simulink model "reduced_pp"  (R2018a)
settings: Solver=VariableStepAuto  StartTime=0.0  StopTime=10.0  RelTol=1e-3
undefined symbols (not defined in the file or in its folder): DiscIntNeverNeededParam
libraries: simulink x24
settings Model: Creator=ishaf  LastModifiedBy=ishaf

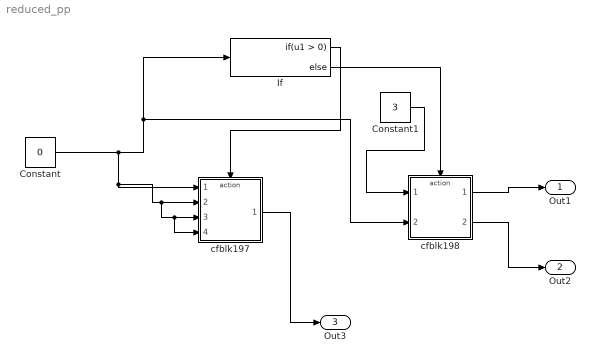
== system reduced_pp ==
  Constant : Constant  Value=0
  Constant1 : Constant  Value=3
  If : If
  cfblk197 : Subsystem  TreatAsAtomicUnit=on
  cfblk198 : Subsystem  TreatAsAtomicUnit=on
  Out1 : Outport
  Out2 : Outport  Port=2
  Out3 : Outport  Port=3
  wires:
  cfblk197/1(cfblk2) -> Out3/1
  Constant/1 -> cfblk197/4(cfblk16), cfblk197/3(cfblk15), cfblk197/2(cfblk14), cfblk197/1(cfblk1), cfblk198/2(cfblk11), If/1
  Constant1/1 -> cfblk198/1(cfblk1)
  cfblk198/1(cfblk2) -> Out1/1
  cfblk198/2(cfblk12) -> Out2/1
  If/1 -> cfblk197/Action
  If/2 -> cfblk198/Action

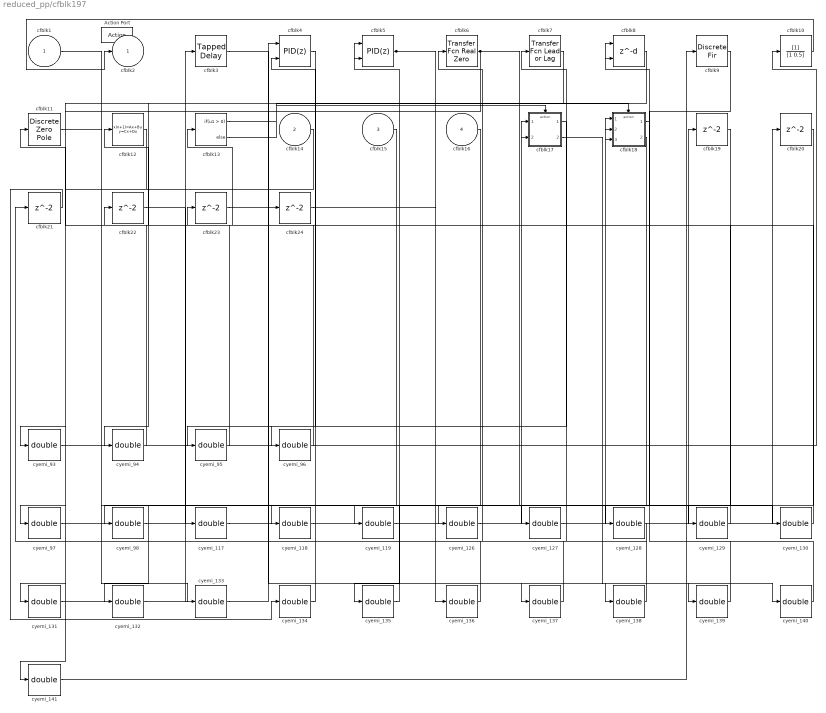
== system reduced_pp/cfblk197 ==
  cfblk1 : Inport
  cfblk14 : Inport  Port=2
  cfblk15 : Inport  Port=3
  cfblk16 : Inport  Port=4
  Action Port : ActionPort  ActionType=then
  cfblk10 : DiscreteFilter
  cfblk11 : DiscreteZeroPole  Poles=[0 0.5]  Gain=1  SampleTime=-1
  cfblk12 : DiscreteStateSpace  SampleTime=-1
  cfblk13 : If  SampleTime=1
  cfblk17 : Subsystem  TreatAsAtomicUnit=on
  cfblk18 : Subsystem  TreatAsAtomicUnit=on
  cfblk{19..24} (6 alike) : Delay
  cfblk3 : simulink/Discrete/Tapped Delay  vinit=0.0  samptime=-1  NumDelays=1  DelayOrder=Oldest  includeCurrent=off
  cfblk4 : simulink/Continuous/PID Controller (2DOF)  Controller=PID  TimeDomain=Discrete-time  SampleTime=-1  IntegratorMethod=Forward Euler  FilterMethod=Forward Euler  Form=Parallel  UseFilter=on  ControllerParametersSource=internal  P=1  I=1  D=0  N=100  b=1  c=1  InitialConditionSource=internal  InitialConditionForIntegrator=0  InitialConditionForFilter=0  ExternalReset=none  LimitOutput=off  UpperSaturationLimit=inf  LowerSaturationLimit=-inf  LinearizeAsGain=off  AntiWindupMode=none  Kb=1  TrackingMode=off  Kt=1  PParamMin=[]  PParamMax=[]  IParamMin=[]  IParamMax=[]  DParamMin=[]  DParamMax=[]  NParamMin=[]  NParamMax=[]  bParamMin=[]  bParamMax=[]  cParamMin=[]  cParamMax=[]  KbParamMin=[]  KbParamMax=[]  KtParamMin=[]  KtParamMax=[]  POutMin=[]  POutMax=[]  IOutMin=[]  IOutMax=[]  DOutMin=[]  DOutMax=[]  NOutMin=[]  NOutMax=[]  bOutMin=[]  bOutMax=[]  cOutMin=[]  cOutMax=[]  KbOutMin=[]  KbOutMax=[]  KtOutMin=[]  KtOutMax=[]  IntegratorOutMin=[]  IntegratorOutMax=[]  FilterOutMin=[]  FilterOutMax=[]  SumOutMin=[]  SumOutMax=[]  Sum1OutMin=[]  Sum1OutMax=[]  Sum2OutMin=[]  Sum2OutMax=[]  Sum3OutMin=[]  Sum3OutMax=[]  SumI1OutMin=[]  SumI1OutMax=[]  SumI2OutMin=[]  SumI2OutMax=[]  SumI3OutMin=[]  SumI3OutMax=[]  SumDOutMin=[]  SumDOutMax=[]  SaturationOutMin=[]  SaturationOutMax=[]  IntegratorContinuousStateAttributes=''  IntegratorStateMustResolveToSignalObject=off  IntegratorRTWStateStorageClass=Auto  FilterContinuousStateAttributes=''  FilterStateMustResolveToSignalObject=off  FilterRTWStateStorageClass=Auto  DifferentiatorICPrevScaledInput=0  DifferentiatorOutMin=[]  DifferentiatorOutMax=[]  FilterDiffOutCoefMin=[]  FilterDiffOutCoefMax=[]  SumDenOutMin=[]  SumDenOutMax=[]  SumNumOutMin=[]  SumNumOutMax=[]  ReciprocalOutMin=[]  ReciprocalOutMax=[]  DivideOutMin=[]  DivideOutMax=[]  TunerSelectOption=Transfer Function Based (PID Tuner App)
  cfblk5 : simulink/Continuous/PID Controller (2DOF)  Controller=PID  TimeDomain=Discrete-time  SampleTime=-1  IntegratorMethod=Forward Euler  FilterMethod=Forward Euler  Form=Parallel  UseFilter=on  ControllerParametersSource=internal  P=1  I=1  D=0  N=100  b=1  c=1  InitialConditionSource=internal  InitialConditionForIntegrator=0  InitialConditionForFilter=0  ExternalReset=none  LimitOutput=off  UpperSaturationLimit=inf  LowerSaturationLimit=-inf  LinearizeAsGain=off  AntiWindupMode=none  Kb=1  TrackingMode=off  Kt=1  PParamMin=[]  PParamMax=[]  IParamMin=[]  IParamMax=[]  DParamMin=[]  DParamMax=[]  NParamMin=[]  NParamMax=[]  bParamMin=[]  bParamMax=[]  cParamMin=[]  cParamMax=[]  KbParamMin=[]  KbParamMax=[]  KtParamMin=[]  KtParamMax=[]  POutMin=[]  POutMax=[]  IOutMin=[]  IOutMax=[]  DOutMin=[]  DOutMax=[]  NOutMin=[]  NOutMax=[]  bOutMin=[]  bOutMax=[]  cOutMin=[]  cOutMax=[]  KbOutMin=[]  KbOutMax=[]  KtOutMin=[]  KtOutMax=[]  IntegratorOutMin=[]  IntegratorOutMax=[]  FilterOutMin=[]  FilterOutMax=[]  SumOutMin=[]  SumOutMax=[]  Sum1OutMin=[]  Sum1OutMax=[]  Sum2OutMin=[]  Sum2OutMax=[]  Sum3OutMin=[]  Sum3OutMax=[]  SumI1OutMin=[]  SumI1OutMax=[]  SumI2OutMin=[]  SumI2OutMax=[]  SumI3OutMin=[]  SumI3OutMax=[]  SumDOutMin=[]  SumDOutMax=[]  SaturationOutMin=[]  SaturationOutMax=[]  IntegratorContinuousStateAttributes=''  IntegratorStateMustResolveToSignalObject=off  IntegratorRTWStateStorageClass=Auto  FilterContinuousStateAttributes=''  FilterStateMustResolveToSignalObject=off  FilterRTWStateStorageClass=Auto  DifferentiatorICPrevScaledInput=0  DifferentiatorOutMin=[]  DifferentiatorOutMax=[]  FilterDiffOutCoefMin=[]  FilterDiffOutCoefMax=[]  SumDenOutMin=[]  SumDenOutMax=[]  SumNumOutMin=[]  SumNumOutMax=[]  ReciprocalOutMin=[]  ReciprocalOutMax=[]  DivideOutMin=[]  DivideOutMax=[]  TunerSelectOption=Transfer Function Based (PID Tuner App)
  cfblk6 : simulink/Discrete/Transfer Fcn Real Zero  ZeroZ=0.75  ICPrevInput=0.0  DoSatur=off
      settings: SourceProductName=Simulink  SourceProductBaseCode=SL
  cfblk7 : simulink/Discrete/Transfer Fcn Lead or Lag  PoleZ=0.95  ZeroZ=0.75  ICPrevOutput=0.0  ICPrevInput=0.0  DoSatur=off
      settings: SourceProductName=Simulink  SourceProductBaseCode=SL
  cfblk8 : Delay  DelayLengthSource=Input port
      settings: InputPortMap=u0,p1
  cfblk9 : DiscreteFir
  cyemi_{93..98,117..119,126..141} (25 alike) : DataTypeConversion  OutDataTypeStr=double
  cfblk2 : Outport
  wires:
  cfblk5/1 -> cyemi_129/1, cyemi_137/1
  cfblk6/1 -> cyemi_130/1, cyemi_131/1
  cfblk10/1 -> cfblk2/1
  cfblk13/1 -> cfblk17/Action
  cfblk13/2 -> cfblk18/Action
  cyemi_93/1 -> cfblk10/1
  cfblk14/1 -> cyemi_93/1
  cyemi_94/1 -> cfblk11/1
  cfblk8/1 -> cyemi_94/1
  cyemi_95/1 -> cfblk12/1
  cfblk17/1(cfblk2) -> cyemi_95/1
  cyemi_96/1 -> cfblk13/1
  cfblk4/1 -> cyemi_96/1
  cyemi_97/1 -> cfblk17/1(cfblk1)
  cfblk7/1 -> cyemi_97/1
  cyemi_98/1 -> cfblk17/2(cfblk16)
  cfblk19/1 -> cyemi_98/1
  cyemi_117/1 -> cfblk18/1(cfblk1)
  cfblk22/1 -> cyemi_117/1
  cyemi_118/1 -> cfblk18/2(cfblk9)
  cfblk20/1 -> cyemi_118/1
  cyemi_119/1 -> cfblk18/3(cfblk10)
  cfblk15/1 -> cyemi_119/1
  cyemi_126/1 -> cfblk19/1
  cfblk9/1 -> cyemi_126/1
  cyemi_127/1 -> cfblk20/1
  cfblk11/1 -> cyemi_127/1
  cyemi_128/1 -> cfblk21/1
  cfblk18/1(cfblk2) -> cyemi_128/1
  cyemi_129/1 -> cfblk22/1
  cyemi_130/1 -> cfblk23/1
  cyemi_131/1 -> cfblk24/1
  cyemi_132/1 -> cfblk3/1
  cfblk16/1 -> cyemi_132/1
  cyemi_133/1 -> cfblk4/1
  cfblk1/1 -> cyemi_133/1
  cyemi_134/1 -> cfblk4/2
  cfblk21/1 -> cyemi_134/1
  cyemi_135/1 -> cfblk5/1
  cfblk18/2(cfblk11) -> cyemi_135/1
  cyemi_136/1 -> cfblk5/2
  cfblk24/1 -> cyemi_136/1
  cyemi_137/1 -> cfblk6/1
  cyemi_138/1 -> cfblk7/1
  cfblk3/1 -> cyemi_138/1
  cyemi_139/1 -> cfblk8/1
  cfblk23/1 -> cyemi_139/1
  cyemi_140/1 -> cfblk8/2
  cfblk17/2(cfblk17) -> cyemi_140/1
  cyemi_141/1 -> cfblk9/1
  cfblk12/1 -> cyemi_141/1

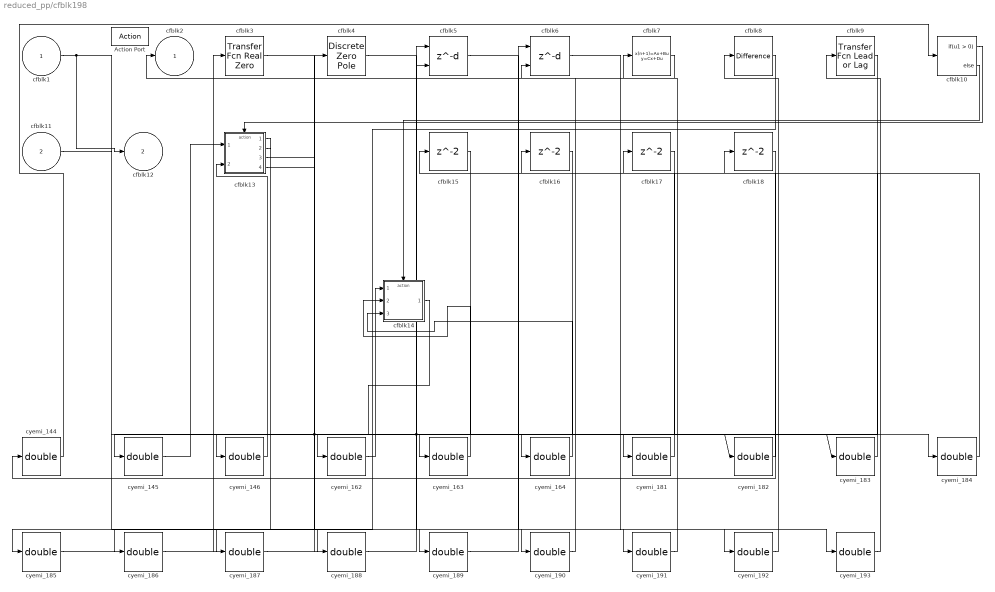
== system reduced_pp/cfblk198 ==
  cfblk1 : Inport
  cfblk11 : Inport  Port=2
  Action Port : ActionPort  ActionType=else
  cfblk10 : If  SampleTime=1
  cfblk13 : Subsystem  TreatAsAtomicUnit=on
  cfblk14 : Subsystem  TreatAsAtomicUnit=on
  cfblk{15..18} (4 alike) : Delay
  cfblk3 : simulink/Discrete/Transfer Fcn Real Zero  ZeroZ=0.75  ICPrevInput=0.0  DoSatur=off
      settings: SourceProductName=Simulink  SourceProductBaseCode=SL
  cfblk4 : DiscreteZeroPole  Poles=[0 0.5]  Gain=1  SampleTime=-1
  cfblk5 : Delay  DelayLengthSource=Input port
      settings: InputPortMap=u0,p1
  cfblk6 : Delay  DelayLengthSource=Input port
      settings: InputPortMap=u0,p1
  cfblk7 : DiscreteStateSpace  SampleTime=-1
  cfblk8 : simulink/Discrete/Difference  ICPrevInput=0.0  OutMin=[]  OutMax=[]  OutDataTypeStr=Inherit: Inherit via back propagation  OutDataType=fixdt(1, 16)  OutScaling=2^-10  DoSatur=off
  cfblk9 : simulink/Discrete/Transfer Fcn Lead or Lag  PoleZ=0.95  ZeroZ=0.75  ICPrevOutput=0.0  ICPrevInput=0.0  DoSatur=off
      settings: SourceProductName=Simulink  SourceProductBaseCode=SL
  cyemi_{144..146,162..164,181..193} (19 alike) : DataTypeConversion  OutDataTypeStr=double
  cfblk2 : Outport
  cfblk12 : Outport  Port=2
  wires:
  cfblk3/1 -> cyemi_182/1, cyemi_189/1
  cfblk7/1 -> cfblk2/1
  cfblk1/1 -> cfblk12/1, cyemi_162/1
  cfblk4/1 -> cyemi_183/1, cyemi_191/1
  cfblk10/1 -> cfblk13/Action
  cfblk10/2 -> cfblk14/Action
  cyemi_144/1 -> cfblk10/1
  cfblk18/1 -> cyemi_144/1
  cyemi_145/1 -> cfblk13/1(cfblk1)
  cfblk14/1(cfblk2) -> cyemi_145/1
  cyemi_146/1 -> cfblk13/2(cfblk13)
  cfblk15/1 -> cyemi_146/1
  cyemi_162/1 -> cfblk14/1(cfblk1)
  cyemi_163/1 -> cfblk14/2(cfblk11)
  cfblk17/1 -> cyemi_163/1
  cyemi_164/1 -> cfblk14/3(cfblk12)
  cfblk16/1 -> cyemi_164/1
  cyemi_181/1 -> cfblk15/1
  cfblk9/1 -> cyemi_181/1
  cyemi_182/1 -> cfblk16/1
  cyemi_183/1 -> cfblk17/1
  cyemi_184/1 -> cfblk18/1
  cfblk13/3(cfblk15) -> cyemi_184/1
  cyemi_185/1 -> cfblk3/1
  cfblk13/1(cfblk2) -> cyemi_185/1
  cyemi_186/1 -> cfblk4/1
  cfblk13/2(cfblk14) -> cyemi_186/1
  cyemi_187/1 -> cfblk5/1
  cfblk8/1 -> cyemi_187/1
  cyemi_188/1 -> cfblk5/2
  cfblk11/1 -> cyemi_188/1
  cyemi_189/1 -> cfblk6/1
  cyemi_190/1 -> cfblk6/2
  cfblk13/4(cfblk16) -> cyemi_190/1
  cyemi_191/1 -> cfblk7/1
  cyemi_192/1 -> cfblk8/1
  cfblk6/1 -> cyemi_192/1
  cyemi_193/1 -> cfblk9/1
  cfblk5/1 -> cyemi_193/1

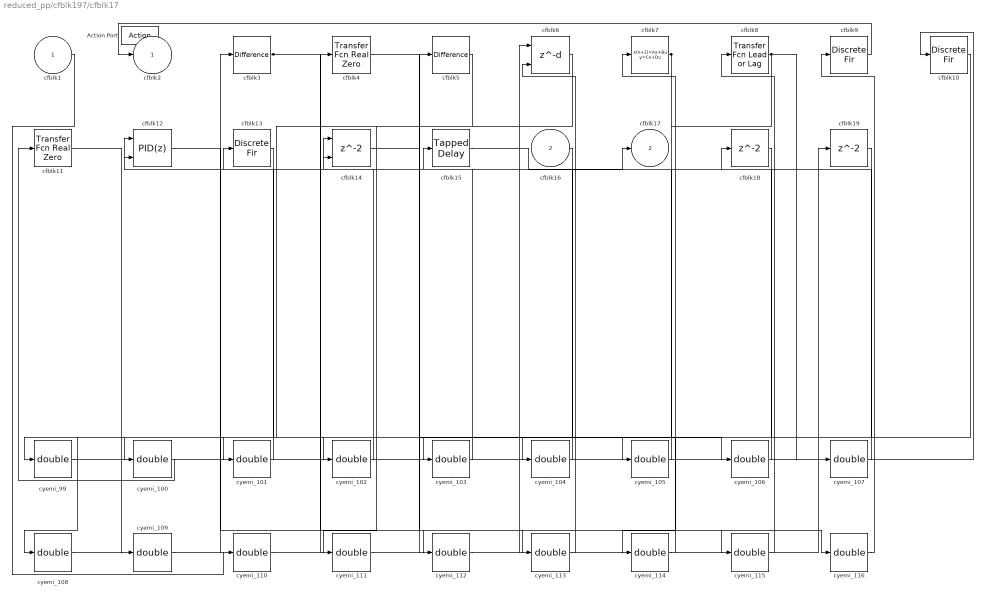
== system reduced_pp/cfblk197/cfblk17 ==
  cfblk1 : Inport
  cfblk16 : Inport  Port=2
  Action Port : ActionPort  ActionType=then
  cfblk10 : DiscreteFir
  cfblk11 : simulink/Discrete/Transfer Fcn Real Zero  ZeroZ=0.75  ICPrevInput=0.0  DoSatur=off
      settings: SourceProductName=Simulink  SourceProductBaseCode=SL
  cfblk12 : simulink/Continuous/PID Controller (2DOF)  Controller=PID  TimeDomain=Discrete-time  SampleTime=-1  IntegratorMethod=Forward Euler  FilterMethod=Forward Euler  Form=Parallel  UseFilter=on  ControllerParametersSource=internal  P=1  I=1  D=0  N=100  b=1  c=1  InitialConditionSource=internal  InitialConditionForIntegrator=0  InitialConditionForFilter=0  ExternalReset=none  LimitOutput=off  UpperSaturationLimit=inf  LowerSaturationLimit=-inf  LinearizeAsGain=off  AntiWindupMode=none  Kb=1  TrackingMode=off  Kt=1  PParamMin=[]  PParamMax=[]  IParamMin=[]  IParamMax=[]  DParamMin=[]  DParamMax=[]  NParamMin=[]  NParamMax=[]  bParamMin=[]  bParamMax=[]  cParamMin=[]  cParamMax=[]  KbParamMin=[]  KbParamMax=[]  KtParamMin=[]  KtParamMax=[]  POutMin=[]  POutMax=[]  IOutMin=[]  IOutMax=[]  DOutMin=[]  DOutMax=[]  NOutMin=[]  NOutMax=[]  bOutMin=[]  bOutMax=[]  cOutMin=[]  cOutMax=[]  KbOutMin=[]  KbOutMax=[]  KtOutMin=[]  KtOutMax=[]  IntegratorOutMin=[]  IntegratorOutMax=[]  FilterOutMin=[]  FilterOutMax=[]  SumOutMin=[]  SumOutMax=[]  Sum1OutMin=[]  Sum1OutMax=[]  Sum2OutMin=[]  Sum2OutMax=[]  Sum3OutMin=[]  Sum3OutMax=[]  SumI1OutMin=[]  SumI1OutMax=[]  SumI2OutMin=[]  SumI2OutMax=[]  SumI3OutMin=[]  SumI3OutMax=[]  SumDOutMin=[]  SumDOutMax=[]  SaturationOutMin=[]  SaturationOutMax=[]  IntegratorContinuousStateAttributes=''  IntegratorStateMustResolveToSignalObject=off  IntegratorRTWStateStorageClass=Auto  FilterContinuousStateAttributes=''  FilterStateMustResolveToSignalObject=off  FilterRTWStateStorageClass=Auto  DifferentiatorICPrevScaledInput=0  DifferentiatorOutMin=[]  DifferentiatorOutMax=[]  FilterDiffOutCoefMin=[]  FilterDiffOutCoefMax=[]  SumDenOutMin=[]  SumDenOutMax=[]  SumNumOutMin=[]  SumNumOutMax=[]  ReciprocalOutMin=[]  ReciprocalOutMax=[]  DivideOutMin=[]  DivideOutMax=[]  TunerSelectOption=Transfer Function Based (PID Tuner App)
  cfblk13 : DiscreteFir
  cfblk14 : Delay  ShowEnablePort=on
      settings: InputPortMap=u0,e6
  cfblk15 : simulink/Discrete/Tapped Delay  vinit=0.0  samptime=-1  NumDelays=1  DelayOrder=Oldest  includeCurrent=off
  cfblk18 : Delay
  cfblk19 : Delay
  cfblk3 : simulink/Discrete/Difference  ICPrevInput=0.0  OutMin=[]  OutMax=[]  OutDataTypeStr=Inherit: Inherit via back propagation  OutDataType=fixdt(1, 16)  OutScaling=2^-10  DoSatur=off
  cfblk4 : simulink/Discrete/Transfer Fcn Real Zero  ZeroZ=0.75  ICPrevInput=0.0  DoSatur=off
      settings: SourceProductName=Simulink  SourceProductBaseCode=SL
  cfblk5 : simulink/Discrete/Difference  ICPrevInput=0.0  OutMin=[]  OutMax=[]  OutDataTypeStr=Inherit: Inherit via back propagation  OutDataType=fixdt(1, 16)  OutScaling=2^-10  DoSatur=off
  cfblk6 : Delay  DelayLengthSource=Input port
      settings: InputPortMap=u0,p1
  cfblk7 : DiscreteStateSpace  SampleTime=-1
  cfblk8 : simulink/Discrete/Transfer Fcn Lead or Lag  PoleZ=0.95  ZeroZ=0.75  ICPrevOutput=0.0  ICPrevInput=0.0  DoSatur=off
      settings: SourceProductName=Simulink  SourceProductBaseCode=SL
  cfblk9 : DiscreteFir
  cyemi_{99..116} (18 alike) : DataTypeConversion  OutDataTypeStr=double
  cfblk2 : Outport
  cfblk17 : Outport  Port=2
  wires:
  cfblk15/1 -> cfblk17/1
  cfblk7/1 -> cyemi_100/1, cyemi_103/1
  cfblk9/1 -> cfblk2/1
  cfblk3/1 -> cyemi_112/1, cyemi_116/1
  cfblk8/1 -> cyemi_105/1, cyemi_107/1
  cyemi_99/1 -> cfblk10/1
  cfblk16/1 -> cyemi_99/1
  cyemi_100/1 -> cfblk11/1
  cyemi_101/1 -> cfblk12/1
  cfblk5/1 -> cyemi_101/1
  cyemi_102/1 -> cfblk12/2
  cfblk18/1 -> cyemi_102/1
  cyemi_103/1 -> cfblk13/1
  cyemi_104/1 -> cfblk14/1
  cfblk10/1 -> cyemi_104/1
  cyemi_105/1 -> cfblk14/2
  cyemi_106/1 -> cfblk15/1
  cfblk14/1 -> cyemi_106/1
  cyemi_107/1 -> cfblk18/1
  cyemi_108/1 -> cfblk19/1
  cfblk13/1 -> cyemi_108/1
  cyemi_109/1 -> cfblk3/1
  cfblk11/1 -> cyemi_109/1
  cyemi_110/1 -> cfblk4/1
  cfblk1/1 -> cyemi_110/1
  cyemi_111/1 -> cfblk5/1
  cfblk6/1 -> cyemi_111/1
  cyemi_112/1 -> cfblk6/1
  cyemi_113/1 -> cfblk6/2
  cfblk4/1 -> cyemi_113/1
  cyemi_114/1 -> cfblk7/1
  cfblk19/1 -> cyemi_114/1
  cyemi_115/1 -> cfblk8/1
  cfblk12/1 -> cyemi_115/1
  cyemi_116/1 -> cfblk9/1

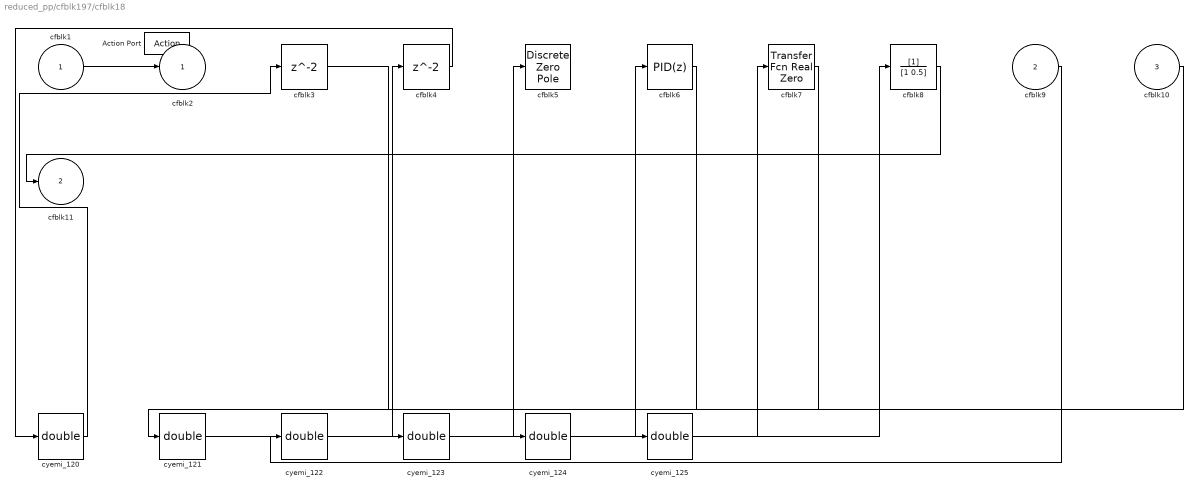
== system reduced_pp/cfblk197/cfblk18 ==
  cfblk1 : Inport
  cfblk9 : Inport  Port=2
  cfblk10 : Inport  Port=3
  Action Port : ActionPort  ActionType=else
  cfblk3 : Delay
  cfblk4 : Delay
  cfblk5 : DiscreteZeroPole  Poles=[0 0.5]  Gain=1  SampleTime=-1
  cfblk6 : simulink/Continuous/PID Controller  Controller=PID  TimeDomain=Discrete-time  SampleTime=-1  IntegratorMethod=Forward Euler  FilterMethod=Forward Euler  Form=Parallel  UseFilter=on  ControllerParametersSource=internal  P=1  I=1  D=0  N=100  InitialConditionSource=internal  InitialConditionForIntegrator=0  InitialConditionForFilter=0  ExternalReset=none  LimitOutput=off  UpperSaturationLimit=inf  LowerSaturationLimit=-inf  LinearizeAsGain=off  AntiWindupMode=none  Kb=1  TrackingMode=off  Kt=1  PParamMin=[]  PParamMax=[]  IParamMin=[]  IParamMax=[]  DParamMin=[]  DParamMax=[]  NParamMin=[]  NParamMax=[]  KbParamMin=[]  KbParamMax=[]  KtParamMin=[]  KtParamMax=[]  POutMin=[]  POutMax=[]  IOutMin=[]  IOutMax=[]  DOutMin=[]  DOutMax=[]  NOutMin=[]  NOutMax=[]  KbOutMin=[]  KbOutMax=[]  KtOutMin=[]  KtOutMax=[]  IntegratorOutMin=[]  IntegratorOutMax=[]  FilterOutMin=[]  FilterOutMax=[]  SumOutMin=[]  SumOutMax=[]  SumI1OutMin=[]  SumI1OutMax=[]  SumI2OutMin=[]  SumI2OutMax=[]  SumI3OutMin=[]  SumI3OutMax=[]  SumDOutMin=[]  SumDOutMax=[]  SaturationOutMin=[]  SaturationOutMax=[]  IntegratorContinuousStateAttributes=''  IntegratorStateMustResolveToSignalObject=off  IntegratorRTWStateStorageClass=Auto  FilterContinuousStateAttributes=''  FilterStateMustResolveToSignalObject=off  FilterRTWStateStorageClass=Auto  DifferentiatorICPrevScaledInput=0  DifferentiatorOutMin=[]  DifferentiatorOutMax=[]  FilterDiffOutCoefMin=[]  FilterDiffOutCoefMax=[]  SumDenOutMin=[]  SumDenOutMax=[]  SumNumOutMin=[]  SumNumOutMax=[]  ReciprocalOutMin=[]  ReciprocalOutMax=[]  DivideOutMin=[]  DivideOutMax=[]  TunerSelectOption=Transfer Function Based (PID Tuner App)
  cfblk7 : simulink/Discrete/Transfer Fcn Real Zero  ZeroZ=0.75  ICPrevInput=0.0  DoSatur=off
      settings: SourceProductName=Simulink  SourceProductBaseCode=SL
  cfblk8 : DiscreteFilter
  cyemi_{120..125} (6 alike) : DataTypeConversion  OutDataTypeStr=double
  cfblk2 : Outport
  cfblk11 : Outport  Port=2
  wires:
  cfblk8/1 -> cfblk11/1
  cfblk1/1 -> cfblk2/1
  cyemi_120/1 -> cfblk3/1
  cfblk4/1 -> cyemi_120/1
  cyemi_121/1 -> cfblk4/1
  cfblk6/1 -> cyemi_121/1
  cyemi_122/1 -> cfblk5/1
  cfblk9/1 -> cyemi_122/1
  cyemi_123/1 -> cfblk6/1
  cfblk10/1 -> cyemi_123/1
  cyemi_124/1 -> cfblk7/1
  cfblk3/1 -> cyemi_124/1
  cyemi_125/1 -> cfblk8/1
  cfblk7/1 -> cyemi_125/1

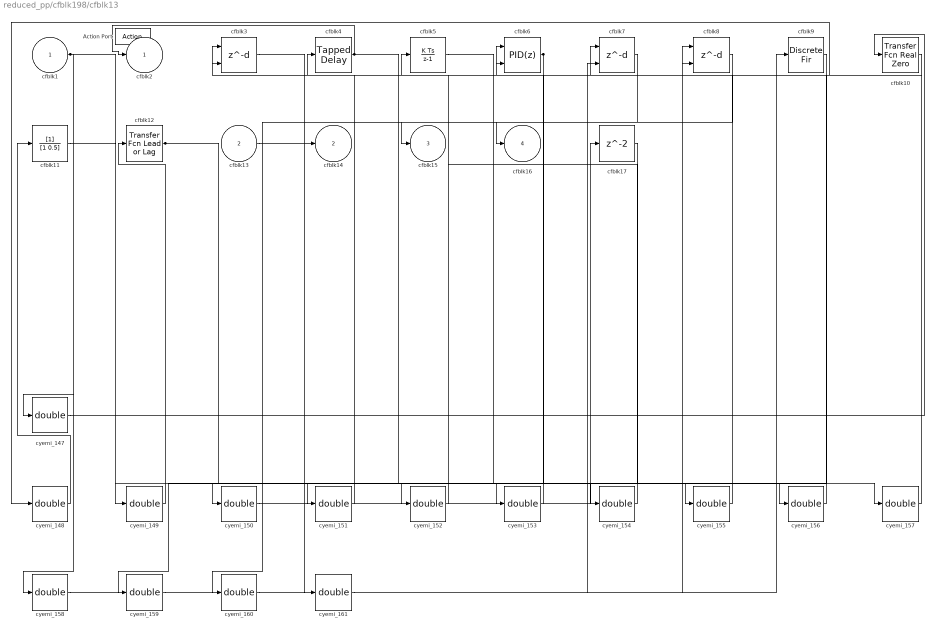
== system reduced_pp/cfblk198/cfblk13 ==
  cfblk1 : Inport
  cfblk13 : Inport  Port=2
  Action Port : ActionPort  ActionType=then
  cfblk10 : simulink/Discrete/Transfer Fcn Real Zero  ZeroZ=0.75  ICPrevInput=0.0  DoSatur=off
      settings: SourceProductName=Simulink  SourceProductBaseCode=SL
  cfblk11 : DiscreteFilter
  cfblk12 : simulink/Discrete/Transfer Fcn Lead or Lag  PoleZ=0.95  ZeroZ=0.75  ICPrevOutput=0.0  ICPrevInput=0.0  DoSatur=off
      settings: SourceProductName=Simulink  SourceProductBaseCode=SL
  cfblk17 : Delay
  cfblk3 : Delay  DelayLengthSource=Input port
      settings: InputPortMap=u0,p1
  cfblk4 : simulink/Discrete/Tapped Delay  vinit=0.0  samptime=-1  NumDelays=1  DelayOrder=Oldest  includeCurrent=off
  cfblk5 : DiscreteIntegrator  SampleTime=-1  ICPrevOutput=DiscIntNeverNeededParam  ICPrevScaledInput=DiscIntNeverNeededParam
  cfblk6 : simulink/Continuous/PID Controller (2DOF)  Controller=PID  TimeDomain=Discrete-time  SampleTime=-1  IntegratorMethod=Forward Euler  FilterMethod=Forward Euler  Form=Parallel  UseFilter=on  ControllerParametersSource=internal  P=1  I=1  D=0  N=100  b=1  c=1  InitialConditionSource=internal  InitialConditionForIntegrator=0  InitialConditionForFilter=0  ExternalReset=none  LimitOutput=off  UpperSaturationLimit=inf  LowerSaturationLimit=-inf  LinearizeAsGain=off  AntiWindupMode=none  Kb=1  TrackingMode=off  Kt=1  PParamMin=[]  PParamMax=[]  IParamMin=[]  IParamMax=[]  DParamMin=[]  DParamMax=[]  NParamMin=[]  NParamMax=[]  bParamMin=[]  bParamMax=[]  cParamMin=[]  cParamMax=[]  KbParamMin=[]  KbParamMax=[]  KtParamMin=[]  KtParamMax=[]  POutMin=[]  POutMax=[]  IOutMin=[]  IOutMax=[]  DOutMin=[]  DOutMax=[]  NOutMin=[]  NOutMax=[]  bOutMin=[]  bOutMax=[]  cOutMin=[]  cOutMax=[]  KbOutMin=[]  KbOutMax=[]  KtOutMin=[]  KtOutMax=[]  IntegratorOutMin=[]  IntegratorOutMax=[]  FilterOutMin=[]  FilterOutMax=[]  SumOutMin=[]  SumOutMax=[]  Sum1OutMin=[]  Sum1OutMax=[]  Sum2OutMin=[]  Sum2OutMax=[]  Sum3OutMin=[]  Sum3OutMax=[]  SumI1OutMin=[]  SumI1OutMax=[]  SumI2OutMin=[]  SumI2OutMax=[]  SumI3OutMin=[]  SumI3OutMax=[]  SumDOutMin=[]  SumDOutMax=[]  SaturationOutMin=[]  SaturationOutMax=[]  IntegratorContinuousStateAttributes=''  IntegratorStateMustResolveToSignalObject=off  IntegratorRTWStateStorageClass=Auto  FilterContinuousStateAttributes=''  FilterStateMustResolveToSignalObject=off  FilterRTWStateStorageClass=Auto  DifferentiatorICPrevScaledInput=0  DifferentiatorOutMin=[]  DifferentiatorOutMax=[]  FilterDiffOutCoefMin=[]  FilterDiffOutCoefMax=[]  SumDenOutMin=[]  SumDenOutMax=[]  SumNumOutMin=[]  SumNumOutMax=[]  ReciprocalOutMin=[]  ReciprocalOutMax=[]  DivideOutMin=[]  DivideOutMax=[]  TunerSelectOption=Transfer Function Based (PID Tuner App)
  cfblk7 : Delay  DelayLengthSource=Input port
      settings: InputPortMap=u0,p1
  cfblk8 : Delay  DelayLengthSource=Input port
      settings: InputPortMap=u0,p1
  cfblk9 : DiscreteFir
  cyemi_{147..161} (15 alike) : DataTypeConversion  OutDataTypeStr=double
  cfblk2 : Outport
  cfblk14 : Outport  Port=2
  cfblk15 : Outport  Port=3
  cfblk16 : Outport  Port=4
  wires:
  cfblk1/1 -> cyemi_147/1, cyemi_155/1, cyemi_158/1
  cfblk4/1 -> cfblk2/1, cyemi_156/1
  cfblk12/1 -> cyemi_154/1, cyemi_161/1
  cfblk13/1 -> cfblk14/1
  cfblk6/1 -> cfblk15/1, cyemi_150/1, cyemi_159/1
  cfblk8/1 -> cfblk16/1
  cyemi_147/1 -> cfblk10/1
  cyemi_148/1 -> cfblk11/1
  cfblk10/1 -> cyemi_148/1
  cyemi_149/1 -> cfblk12/1
  cfblk11/1 -> cyemi_149/1
  cyemi_150/1 -> cfblk17/1
  cyemi_151/1 -> cfblk3/1
  cfblk9/1 -> cyemi_151/1
  cyemi_152/1 -> cfblk3/2
  cfblk17/1 -> cyemi_152/1
  cyemi_153/1 -> cfblk4/1
  cfblk3/1 -> cyemi_153/1
  cyemi_154/1 -> cfblk5/1
  cyemi_155/1 -> cfblk6/1
  cyemi_156/1 -> cfblk6/2
  cyemi_157/1 -> cfblk7/1
  cfblk5/1 -> cyemi_157/1
  cyemi_158/1 -> cfblk7/2
  cyemi_159/1 -> cfblk8/1
  cyemi_160/1 -> cfblk8/2
  cfblk7/1 -> cyemi_160/1
  cyemi_161/1 -> cfblk9/1

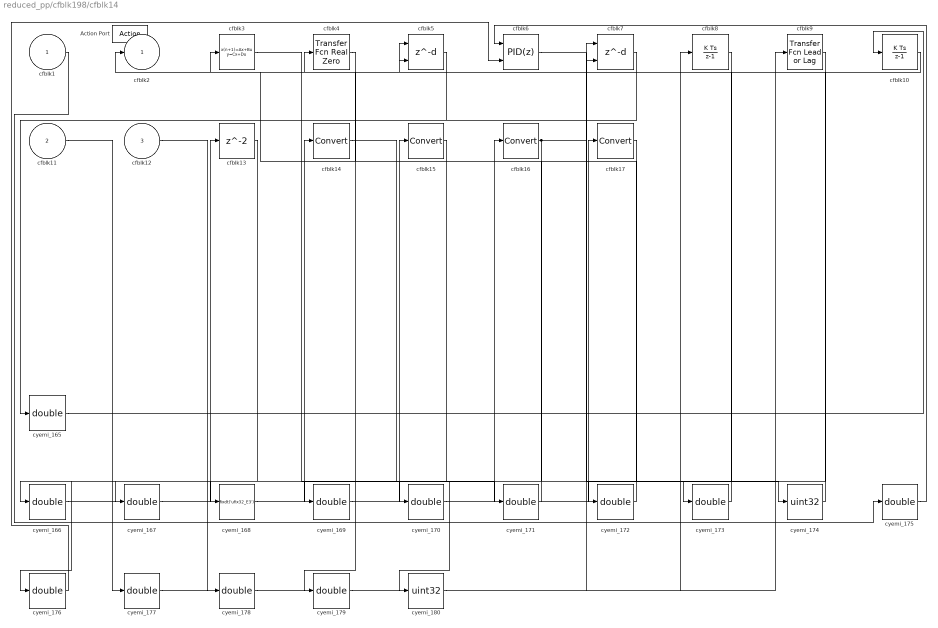
== system reduced_pp/cfblk198/cfblk14 ==
  cfblk1 : Inport
  cfblk11 : Inport  Port=2
  cfblk12 : Inport  Port=3
  Action Port : ActionPort  ActionType=else
  cfblk10 : DiscreteIntegrator  SampleTime=-1  ICPrevOutput=DiscIntNeverNeededParam  ICPrevScaledInput=DiscIntNeverNeededParam
  cfblk13 : Delay
  cfblk{14..17} (4 alike) : DataTypeConversion
  cfblk3 : DiscreteStateSpace  SampleTime=-1
  cfblk4 : simulink/Discrete/Transfer Fcn Real Zero  ZeroZ=0.75  ICPrevInput=0.0  DoSatur=off
      settings: SourceProductName=Simulink  SourceProductBaseCode=SL
  cfblk5 : Delay  DelayLengthSource=Input port
      settings: InputPortMap=u0,p1
  cfblk6 : simulink/Continuous/PID Controller (2DOF)  Controller=PID  TimeDomain=Discrete-time  SampleTime=-1  IntegratorMethod=Forward Euler  FilterMethod=Forward Euler  Form=Parallel  UseFilter=on  ControllerParametersSource=internal  P=1  I=1  D=0  N=100  b=1  c=1  InitialConditionSource=internal  InitialConditionForIntegrator=0  InitialConditionForFilter=0  ExternalReset=none  LimitOutput=off  UpperSaturationLimit=inf  LowerSaturationLimit=-inf  LinearizeAsGain=off  AntiWindupMode=none  Kb=1  TrackingMode=off  Kt=1  PParamMin=[]  PParamMax=[]  IParamMin=[]  IParamMax=[]  DParamMin=[]  DParamMax=[]  NParamMin=[]  NParamMax=[]  bParamMin=[]  bParamMax=[]  cParamMin=[]  cParamMax=[]  KbParamMin=[]  KbParamMax=[]  KtParamMin=[]  KtParamMax=[]  POutMin=[]  POutMax=[]  IOutMin=[]  IOutMax=[]  DOutMin=[]  DOutMax=[]  NOutMin=[]  NOutMax=[]  bOutMin=[]  bOutMax=[]  cOutMin=[]  cOutMax=[]  KbOutMin=[]  KbOutMax=[]  KtOutMin=[]  KtOutMax=[]  IntegratorOutMin=[]  IntegratorOutMax=[]  FilterOutMin=[]  FilterOutMax=[]  SumOutMin=[]  SumOutMax=[]  Sum1OutMin=[]  Sum1OutMax=[]  Sum2OutMin=[]  Sum2OutMax=[]  Sum3OutMin=[]  Sum3OutMax=[]  SumI1OutMin=[]  SumI1OutMax=[]  SumI2OutMin=[]  SumI2OutMax=[]  SumI3OutMin=[]  SumI3OutMax=[]  SumDOutMin=[]  SumDOutMax=[]  SaturationOutMin=[]  SaturationOutMax=[]  IntegratorContinuousStateAttributes=''  IntegratorStateMustResolveToSignalObject=off  IntegratorRTWStateStorageClass=Auto  FilterContinuousStateAttributes=''  FilterStateMustResolveToSignalObject=off  FilterRTWStateStorageClass=Auto  DifferentiatorICPrevScaledInput=0  DifferentiatorOutMin=[]  DifferentiatorOutMax=[]  FilterDiffOutCoefMin=[]  FilterDiffOutCoefMax=[]  SumDenOutMin=[]  SumDenOutMax=[]  SumNumOutMin=[]  SumNumOutMax=[]  ReciprocalOutMin=[]  ReciprocalOutMax=[]  DivideOutMin=[]  DivideOutMax=[]  TunerSelectOption=Transfer Function Based (PID Tuner App)
  cfblk7 : Delay  DelayLengthSource=Input port
      settings: InputPortMap=u0,p1
  cfblk8 : DiscreteIntegrator  SampleTime=-1  ICPrevOutput=DiscIntNeverNeededParam  ICPrevScaledInput=DiscIntNeverNeededParam
  cfblk9 : simulink/Discrete/Transfer Fcn Lead or Lag  PoleZ=0.95  ZeroZ=0.75  ICPrevOutput=0.0  ICPrevInput=0.0  DoSatur=off
      settings: SourceProductName=Simulink  SourceProductBaseCode=SL
  cyemi_{165..167,169..173,175..179} (13 alike) : DataTypeConversion  OutDataTypeStr=double
  cyemi_168 : DataTypeConversion  OutDataTypeStr=fixdt('ufix32_E3')
  cyemi_174 : DataTypeConversion  OutDataTypeStr=uint32
  cyemi_180 : DataTypeConversion  OutDataTypeStr=uint32
  cfblk2 : Outport
  wires:
  cfblk10/1 -> cfblk2/1
  cfblk16/1 -> cyemi_174/1, cyemi_180/1
  cyemi_165/1 -> cfblk10/1
  cfblk5/1 -> cyemi_165/1
  cyemi_166/1 -> cfblk13/1
  cfblk15/1 -> cyemi_166/1
  cyemi_167/1 -> cfblk14/1
  cfblk13/1 -> cyemi_167/1
  cyemi_168/1 -> cfblk15/1
  cfblk9/1 -> cyemi_168/1
  cyemi_169/1 -> cfblk16/1
  cfblk4/1 -> cyemi_169/1
  cyemi_170/1 -> cfblk17/1
  cfblk3/1 -> cyemi_170/1
  cyemi_171/1 -> cfblk3/1
  cfblk14/1 -> cyemi_171/1
  cyemi_172/1 -> cfblk4/1
  cfblk17/1 -> cyemi_172/1
  cyemi_173/1 -> cfblk5/1
  cfblk6/1 -> cyemi_173/1
  cyemi_174/1 -> cfblk5/2
  cyemi_175/1 -> cfblk6/1
  cfblk1/1 -> cyemi_175/1
  cyemi_176/1 -> cfblk6/2
  cfblk8/1 -> cyemi_176/1
  cyemi_177/1 -> cfblk7/1
  cfblk11/1 -> cyemi_177/1
  cyemi_178/1 -> cfblk7/2
  cfblk12/1 -> cyemi_178/1
  cyemi_179/1 -> cfblk8/1
  cfblk7/1 -> cyemi_179/1
  cyemi_180/1 -> cfblk9/1
